simulink model "ballistic_flight_phase"  (R2015a)
settings: Solver=ode45  StartTime=0.0  StopTime=t_max  RelTol=1e-3
values from neighbouring files (symbols this model uses):
  q1_init = 5*pi/6    (= 2.61799387799)    [main.m]
  q2_init = pi + asin(l1/(2*l2))    [main.m]
  tau = -40    [main.m]
  tau_sat = 180    [main.m]
settings Model: Creator=root  LastModifiedBy=root

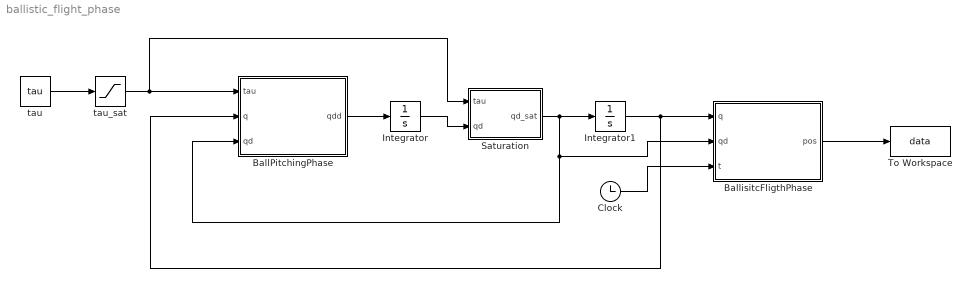
== system ballistic_flight_phase ==
  BallPitchingPhase : MATLAB Function  TreatAsAtomicUnit=on
  BallisitcFligthPhase : MATLAB Function  TreatAsAtomicUnit=on
  Clock : Clock
  Integrator : Integrator  InitialCondition=[0;0]
  Integrator1 : Integrator  InitialCondition=[q1_init;q2_init]
  Saturation : MATLAB Function  TreatAsAtomicUnit=on
  To Workspace : ToWorkspace  VariableName=data  SaveFormat=Timeseries  SampleTime=-1
  tau : Constant  Value=tau
  tau_sat : Saturate  UpperLimit=tau_sat  LowerLimit=-tau_sat
  wires:
  BallPitchingPhase/1(qdd) -> Integrator/1
  Integrator1/1 -> BallPitchingPhase/2(q), BallisitcFligthPhase/1(q)
  Clock/1 -> BallisitcFligthPhase/3(t)
  BallisitcFligthPhase/1(pos) -> To Workspace/1
  tau/1 -> tau_sat/1
  tau_sat/1 -> BallPitchingPhase/1(tau), Saturation/1(tau)
  Integrator/1 -> Saturation/2(qd)
  Saturation/1(qd_sat) -> BallisitcFligthPhase/2(qd), BallPitchingPhase/3(qd), Integrator1/1

== matlab function ballistic_flight_phase/BallisitcFligthPhase ==
  data: q input; qd input; t input; pos output
function pos = fcn(q, qd, t)
    persistent first transition l1 l2 p0 v0 g
    
    if isempty(first),
        l1 = 0.3;
        l2 = 0.542;
        g = 9.81;
        first = 1;
        transition = 0;
        p0 = [0;0];
        v0 = [0;0];
    end
    
    q1 = q(1);
    q2 = q(2);
    qd1 = qd(1);
    qd2 = qd(2);
    
    pp = [l1*cos(q1)+l2*cos(q2); l1*sin(q1)+l2*sin(q2)];
    vp = [-l1*qd1*sin(q1)-l2*qd2*sin(q2); l1*qd1*cos(q1)+l2*qd2*cos(q2)];
    
    if pp(1) >= -0.1  && transition == 0,
       p0 = pp;
       v0 = vp;
       disp(p0)
       disp(v0)
       transition = 1;
    end
    
    if transition == 1
        x = v0(1)*t + p0(1);
        y = v0(2)*t + p0(2)-g/2*t^2;
        if y <= 0
            pos = [x;0];
        else
            pos = [x;y];
        end
    else
        pos = pp;
    end
end

== matlab function ballistic_flight_phase/BallPitchingPhase ==
  data: tau input; q input; qdd output; qd input
function qdd = fcn(tau, q, qd)
    persistent first l1 l2 m1 m2 l1c l2c I1 I2 k2 mB g
    
    if isempty(first),
        l1 = 0.3;
        l2 = 0.542;
        m1 = 2.934;
        m2 = 1.1022;
        l1c = 0.2071;
        l2c = 0.2717;
        I1 = 0.2067;
        I2 = 0.1362;
        k2 = 14.1543;
        mB = 0.064;
        g = 9.81;
        first = 1;
    end
    q1 = q(1);
    q2 = q(2);
    qd1 = qd(1);
    qd2 = qd(2);
    
    m11 = m1*l1c^2+(m2+mB)*l1^2+I1; 
    m12 = (m2+mB)*l1*l2*cos(q1-q2);
    m21 = (m2+mB)*l1*l2*cos(q1-q2);
    m22 = I2 + (m2+mB)*l2^2;
    c11 = 0;
    c12 = (m2+mB)*l1*l2*sin(q1-q2)*qd2;
    c21 = -(m2+mB)*l1*l2*sin(q1-q2)*qd1;
    c22 = 0;
    g11 = m1*g*l1c*cos(q1)+(m2+mB)*g*l1*cos(q1);
    g22 = m2*g*l2c*cos(q2)+mB*g*l2*cos(q2);
    k11 = -k2*(q2-q1);  
    k22 = k2*(q2-q1);
    
    M = [m11 m12; m21 m22];
    C = [c11 c12; c21 c22];
    G = [g11; g22];
    K = [k11; k22];
    u = [tau; 0];

qdd = M\(u-C*qd-G-K);

== matlab function ballistic_flight_phase/Saturation ==
  data: tau input; qd_sat output; qd input
function qd_sat = fcn(tau, qd)
qd1_SAT = 3.787;
pwr_SAT = 270;

qd1 = qd(1);
qd2 = qd(2);

if abs(qd1) > qd1_SAT
    dq1 = sign(qd1)*qd1_SAT;
end

if abs(tau*qd1) > pwr_SAT
    dq1 = sign(qd1)*pwr_SAT/abs(tau);
end

qd_sat = [qd1; qd2];
